simulink model "dpd_top"  (R2025b)
settings: Solver=FixedStepDiscrete  StartTime=0.0  StopTime=length(tx_bb)*Ts  FixedStep=Ts  RelTol=1e-3
undefined symbols (not defined in the file): Ts
settings Model: Creator=zhuyong  LastModifiedBy=zhuyong

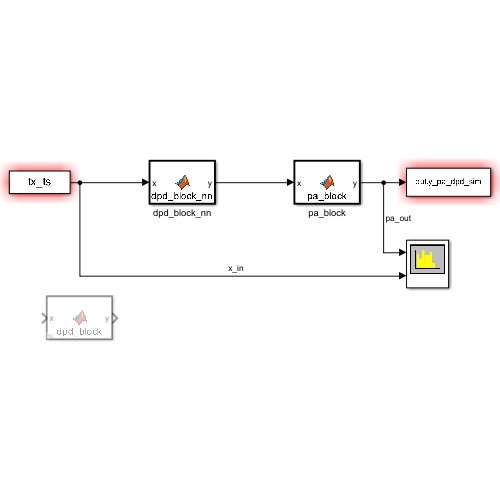
[thumbnail: Simulink's stored preview of the top-level diagram]
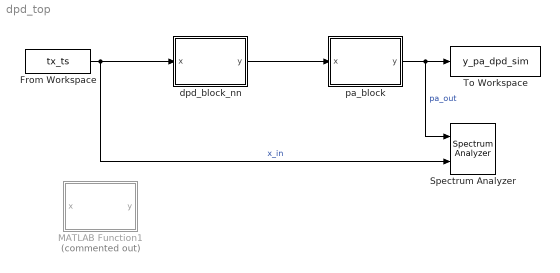
== system dpd_top ==
  From Workspace : FromWorkspace  VariableName=tx_ts  SampleTime=-1
  MATLAB Function1 : MATLAB Function  Commented=on  TreatAsAtomicUnit=on
  Spectrum Analyzer : SpectrumAnalyzer  NumInputPorts=2  WindowPosition=[0.000000,36.000000,1536.000000,793.000000,]  ScopeFrameLocation=window  SampleRateSource=Property  SampleRate=Fs  WindowInvariantSamplesPerUpdate=on  Span=122880000  StartFrequency=-61440000  StopFrequency=61440000  MaximizeAxes=Off  YLimits=[-43.5614 13.4655]  ShowLegend=on
  To Workspace : ToWorkspace  VariableName=y_pa_dpd_sim  SampleTime=Ts
  dpd_block_nn : MATLAB Function  TreatAsAtomicUnit=on
  pa_block : MATLAB Function  TreatAsAtomicUnit=on
  wires:
  From Workspace/1 -> dpd_block_nn/1(x), Spectrum Analyzer/2  "x_in"
  pa_block/1(y) -> To Workspace/1, Spectrum Analyzer/1  "pa_out"
  dpd_block_nn/1(y) -> pa_block/1(x)

== matlab function dpd_top/pa_block ==
  data: x input; y output
function y = pa_block(x)
%#codegen
% 在线记忆多项式 PA 模型（与 pa_memory_poly 一致的形式）
% x、y：标量复数输入输出（逐样本处理）

persistent buf;
if isempty(buf)
    buf = complex(zeros(3,1));   % K = 3 tap 记忆
end

% 更新 buffer：buf(1) 保存当前样本，buf(2)、buf(3) 为过去样本
buf = [x; buf(1:end-1)];

% 系数（与 pa_memory_poly 中保持一致或相近）
a11 = 1.0;   a12 = -0.05;  a13 = 0.02;   % 1 阶
a31 = 0.8;   a32 = -0.04;  a33 = 0.015;  % 3 阶
a51 = 0.3;   a52 = -0.02;  a53 = 0.010;  % 5 阶

acc = complex(0,0);
for k = 1:3
    xnk = buf(k);
    r   = abs(xnk);
    acc = acc ...
        + eval1(a11,a12,a13,k) * xnk ...
        + eval1(a31,a32,a33,k) * xnk * (r^2) ...
        + eval1(a51,a52,a53,k) * xnk * (r^4);
end

y = acc;

% 内部小函数：根据 tap 选择对应的系数
function c = eval1(c1,c2,c3,idx)
    if idx == 1
        c = c1;
    elseif idx == 2
        c = c2;
    else
        c = c3;
    end
end

end

== matlab function dpd_top/dpd_block_nn ==
  data: x input; y output
function y = dpd_block_nn(x)
%#codegen
% dpd_block_nn  基于已训练 NN 的预失真器（仿真专用）
%
% 输入：
%   x : 当前时刻的理想基带输入（complex double 标量）
% 输出：
%   y : 送入 PA 的预失真输出（complex double 标量）

% 声明外部预测函数为 extrinsic（只在仿真中由 MATLAB 执行）
coder.extrinsic('nn_dpd_predict');

% 记忆阶数（与训练时的 K 一致，这里直接写死）
K = 3;

% 持久化记忆 buffer（K×1 复数）
persistent buf
if isempty(buf)
    buf = complex(zeros(K,1));
end

% 确保 x 为 complex double
x = complex(x);

% 更新记忆：buf(1) = x[n], buf(2..K) = x[n-1..n-K+1]
buf = [x; buf(1:end-1)];

% 构造特征向量 feat: 1×(2K)
feat = zeros(1, 2*K);   % double
for k = 1:K
    feat(2*k-1) = real(buf(k));
    feat(2*k)   = imag(buf(k));
end

% 预分配 y_pred，显式告诉代码生成：这是 1×2 double
y_pred = zeros(1,2);
% 调用外部 NN 预测函数
y_pred = nn_dpd_predict(feat);   % extrinsic 调用

% 组合为复数输出
y = complex(y_pred(1), y_pred(2));

end

== matlab function dpd_top/MATLAB Function1 ==
  data: x input; y output
function y = dpd_block(x)
%#codegen
y = x;
end
